simulink model "HANcoder_E407_TTA_Controller_v3_2"  (R2018b)
settings: Solver=FixedStepDiscrete  StartTime=0.0  StopTime=1  FixedStep=0.01  RelTol=1e-3
PreLoadFcn:
  | librarySetup
  | eval([bdroot,'_startup']) %Calling [modelName]_startup.m
undefined symbols (not defined in the file): A0, A1, A2, A3, A4, Backup_Board, basic_cycle_duration_bc0, basic_cycle_duration_bc1, comm_delay_estimation1, comm_delay_estimation2, COMM_Period, COMM_Phase1, COMM_Phase2, COMM_Phase_init1, COMM_Phase_init2, COMP_duration, CON2, CON4, Controller1_Board, Controller2_Board, Controller3_Board, D10, D12, D13, D8, D9, delta_a_set, delta_f_set, delta_max, delta_min, delta_precision, e_width, frequency_IRQ, HANtuneOverride, hardware_granularity, I_a, I_f, idle_time_init, Input_Gen_Board, LA_Clock_Gr, LA_COMM_dly, LA_COMM_Err, LA_E_Desync, LA_MEX_Flag, LA_Task_Act, m_v, Master_Role, matrix_cycle_duration, matrix_rows, max_desync, max_num_msgs_CAN1, max_num_msgs_CAN2, min_desync, OutControl1_ID, OutControl2_ID, OutEmulator_ID, R_al, R_ar, R_fl, R_fr ... (+80)
libraries: hdlsllib x434, HANcoder_STM32_Target x28, simulink x3, simulink_extras x1
(part 14 of 31)

== system HANcoder_E407_TTA_Controller_v3_2/HANcoder STM32 Target - E407-STM32 algorithm/TTA CAN System/TTA System/Matrix Cycle Manager/Controller Matrix Cycle/controller basic cycle 1/COMP Task - TMR/TMR_load_msgs_1 ==
  note: STEP 1 - Gather Output1 and Output2 messages
  note: Logic Analyzer - DEBUG
      | LT Update COMP task
      | activation
  note: Logic Analyzer - DEBUG
  Enable : EnablePort
  Bus Selector : BusSelector  OutputSignals=Buffer_2,Buffer_3,Buffer_4,Buffer_5,Buffer_6,Buffer_7
  Constant{9..12} (4 alike) : Constant  Value=torque_precision
  Constant8 : Constant  Priority=28  OutDataTypeStr=boolean
  Data Store Read : DataStoreRead  DataStoreName=output_control1_msg
  Data Store Write : DataStoreWrite  Priority=1  DataStoreName=tau_fr_out1
  Data Store Write1 : DataStoreWrite  Priority=2  DataStoreName=tau_fl_out1
  Data Store Write19 : DataStoreWrite  Priority=29  DataStoreName=Toggle_Pin_A0
  Data Store Write2 : DataStoreWrite  Priority=3  DataStoreName=tau_ar_out1
  Data Store Write3 : DataStoreWrite  Priority=4  DataStoreName=tau_al_out1
  Data Store Write4 : DataStoreWrite  Priority=5  DataStoreName=set_miss_out1
  Data Store Write5 : DataStoreWrite  Priority=6  DataStoreName=sensor_miss_out1
  uint8_2float : Subsystem
  uint8_2float1 : Subsystem
  uint8_2float2 : Subsystem
  uint8_2float3 : Subsystem
  wires:
  Data Store Read/1 -> Bus Selector/1
  Bus Selector/1 -> uint8_2float/2(value)  "<Buffer_2>"
  Bus Selector/2 -> uint8_2float1/2(value)  "<Buffer_3>"
  Bus Selector/3 -> uint8_2float2/2(value)  "<Buffer_4>"
  Bus Selector/4 -> uint8_2float3/2(value)  "<Buffer_5>"
  Bus Selector/5 -> Data Store Write4/1  "<Buffer_6>"
  Bus Selector/6 -> Data Store Write5/1  "<Buffer_7>"
  Constant8/1 -> Data Store Write19/1
  Constant9/1 -> uint8_2float/1(precision)
  uint8_2float/1(decoded) -> Data Store Write/1  "torque_fr_out1_s"
  Constant10/1 -> uint8_2float1/1(precision)
  Constant11/1 -> uint8_2float2/1(precision)
  Constant12/1 -> uint8_2float3/1(precision)
  uint8_2float1/1(decoded) -> Data Store Write1/1  "torque_fl_out1_s"
  uint8_2float2/1(decoded) -> Data Store Write2/1  "torque_ar_out1_s"
  uint8_2float3/1(decoded) -> Data Store Write3/1  "torque_al_out1_s"

== system HANcoder_E407_TTA_Controller_v3_2/HANcoder STM32 Target - E407-STM32 algorithm/TTA CAN System/TTA System/Matrix Cycle Manager/Controller Matrix Cycle/controller basic cycle 1/COMP Task - TMR/TMR_load_msgs_2 ==
  note: Logic Analyzer - DEBUG
  note: Logic Analyzer - DEBUG
      | LT Update COMP task
      | activation
  note: STEP 1 - Gather Output1 and Output2 messages
  Enable : EnablePort
  Bus Selector1 : BusSelector  OutputSignals=Buffer_2,Buffer_3,Buffer_4,Buffer_5,Buffer_6,Buffer_7
  Constant{13..16} (4 alike) : Constant  Value=torque_precision
  Constant8 : Constant  Priority=28  OutDataTypeStr=boolean
  Data Store Read1 : DataStoreRead  DataStoreName=output_control2_msg
  Data Store Write10 : DataStoreWrite  Priority=11  DataStoreName=set_miss_out2
  Data Store Write11 : DataStoreWrite  Priority=12  DataStoreName=sensor_miss_out2
  Data Store Write19 : DataStoreWrite  Priority=29  DataStoreName=Toggle_Pin_A0
  Data Store Write6 : DataStoreWrite  Priority=7  DataStoreName=tau_fr_out2
  Data Store Write7 : DataStoreWrite  Priority=8  DataStoreName=tau_fl_out2
  Data Store Write8 : DataStoreWrite  Priority=9  DataStoreName=tau_ar_out2
  Data Store Write9 : DataStoreWrite  Priority=10  DataStoreName=tau_al_out2
  uint8_2float4 : Subsystem
  uint8_2float5 : Subsystem
  uint8_2float6 : Subsystem
  uint8_2float7 : Subsystem
  wires:
  uint8_2float4/1(decoded) -> Data Store Write6/1  "torque_fr_out2_s"
  uint8_2float5/1(decoded) -> Data Store Write7/1  "torque_fl_out2_s"
  uint8_2float6/1(decoded) -> Data Store Write8/1  "torque_ar_out2_s"
  uint8_2float7/1(decoded) -> Data Store Write9/1  "torque_al_out2_s"
  Constant16/1 -> uint8_2float7/1(precision)
  Constant15/1 -> uint8_2float6/1(precision)
  Constant14/1 -> uint8_2float5/1(precision)
  Bus Selector1/1 -> uint8_2float4/2(value)  "<Buffer_2>"
  Constant13/1 -> uint8_2float4/1(precision)
  Constant8/1 -> Data Store Write19/1
  Data Store Read1/1 -> Bus Selector1/1
  Bus Selector1/2 -> uint8_2float5/2(value)  "<Buffer_3>"
  Bus Selector1/3 -> uint8_2float6/2(value)  "<Buffer_4>"
  Bus Selector1/4 -> uint8_2float7/2(value)  "<Buffer_5>"
  Bus Selector1/5 -> Data Store Write10/1  "<Buffer_6>"
  Bus Selector1/6 -> Data Store Write11/1  "<Buffer_7>"

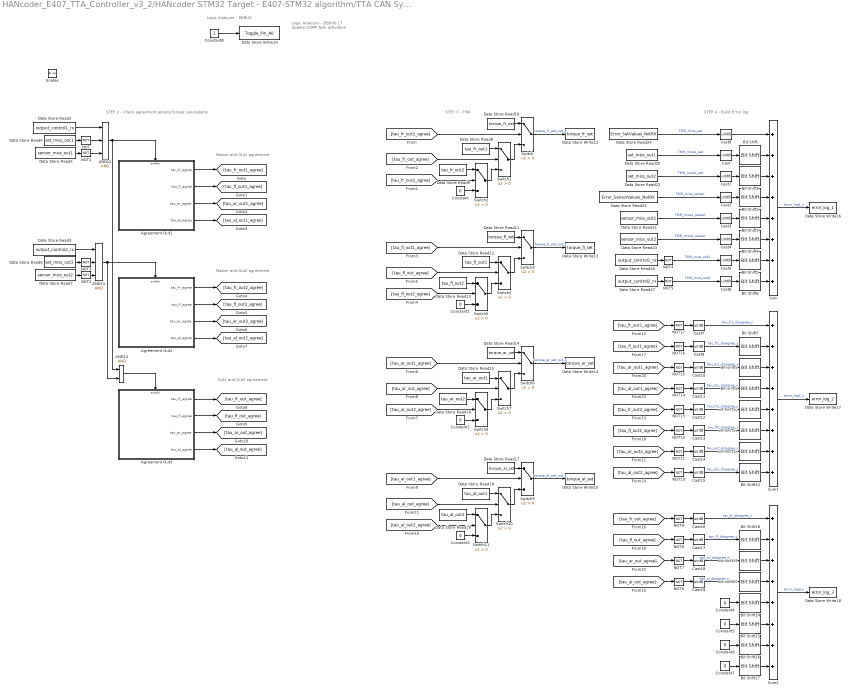
== system HANcoder_E407_TTA_Controller_v3_2/HANcoder STM32 Target - E407-STM32 algorithm/TTA CAN System/TTA System/Matrix Cycle Manager/Controller Matrix Cycle/controller basic cycle 1/COMP Task - TMR/TMR_main ==
  note: Master and Out1 agreement
  note: Logic Analyzer - DEBUG
  note: Logic Analyzer - DEBUG
      | LT Update COMP task
      | activation
  note: STEP 2 - Check agreement among torque calculations
  note: STEP 3 - TMR
  note: STEP 4 - Build Error log
  note: Master and Out2 agreement
  note: Out1 and Out2 agreement
  Enable : EnablePort
  AND12 : Logic  Inputs=3  IconShape=distinctive  AllPortsSameDT=off  OutDataTypeStr=boolean
  AND13 : Logic  Inputs=3  IconShape=distinctive  AllPortsSameDT=off  OutDataTypeStr=boolean
  AND14 : Logic  IconShape=distinctive  AllPortsSameDT=off  OutDataTypeStr=boolean
  Agreement Out1 : Subsystem  Priority=20  TreatAsAtomicUnit=on
  Agreement Out2 : Subsystem  Priority=21  TreatAsAtomicUnit=on
  Agreement Out3 : Subsystem  Priority=22  TreatAsAtomicUnit=on
  Bit Shift : hdlsllib/Logic and Bit Operations/Bit Shift  mode=Shift Left Logical  N=1
      settings: SourceProductName=HDL Coder  SourceProductBaseCode=HD
  Bit Shift1 : hdlsllib/Logic and Bit Operations/Bit Shift  mode=Shift Left Logical  N=2
      settings: SourceProductName=HDL Coder  SourceProductBaseCode=HD
  Bit Shift10 : hdlsllib/Logic and Bit Operations/Bit Shift  mode=Shift Left Logical  N=4
      settings: SourceProductName=HDL Coder  SourceProductBaseCode=HD
  Bit Shift11 : hdlsllib/Logic and Bit Operations/Bit Shift  mode=Shift Left Logical  N=5
      settings: SourceProductName=HDL Coder  SourceProductBaseCode=HD
  Bit Shift12 : hdlsllib/Logic and Bit Operations/Bit Shift  mode=Shift Left Logical  N=6
      settings: SourceProductName=HDL Coder  SourceProductBaseCode=HD
  Bit Shift13 : hdlsllib/Logic and Bit Operations/Bit Shift  mode=Shift Left Logical  N=7
      settings: SourceProductName=HDL Coder  SourceProductBaseCode=HD
  Bit Shift14 : hdlsllib/Logic and Bit Operations/Bit Shift  mode=Shift Left Logical  N=4
      settings: SourceProductName=HDL Coder  SourceProductBaseCode=HD
  Bit Shift15 : hdlsllib/Logic and Bit Operations/Bit Shift  mode=Shift Left Logical  N=5
      settings: SourceProductName=HDL Coder  SourceProductBaseCode=HD
  Bit Shift16 : hdlsllib/Logic and Bit Operations/Bit Shift  mode=Shift Left Logical  N=6
      settings: SourceProductName=HDL Coder  SourceProductBaseCode=HD
  Bit Shift17 : hdlsllib/Logic and Bit Operations/Bit Shift  mode=Shift Left Logical  N=7
      settings: SourceProductName=HDL Coder  SourceProductBaseCode=HD
  Bit Shift18 : hdlsllib/Logic and Bit Operations/Bit Shift  mode=Shift Left Logical  N=1
      settings: SourceProductName=HDL Coder  SourceProductBaseCode=HD
  Bit Shift19 : hdlsllib/Logic and Bit Operations/Bit Shift  mode=Shift Left Logical  N=2
      settings: SourceProductName=HDL Coder  SourceProductBaseCode=HD
  Bit Shift2 : hdlsllib/Logic and Bit Operations/Bit Shift  mode=Shift Left Logical  N=3
      settings: SourceProductName=HDL Coder  SourceProductBaseCode=HD
  Bit Shift20 : hdlsllib/Logic and Bit Operations/Bit Shift  mode=Shift Left Logical  N=3
      settings: SourceProductName=HDL Coder  SourceProductBaseCode=HD
  Bit Shift3 : hdlsllib/Logic and Bit Operations/Bit Shift  mode=Shift Left Logical  N=4
      settings: SourceProductName=HDL Coder  SourceProductBaseCode=HD
  Bit Shift4 : hdlsllib/Logic and Bit Operations/Bit Shift  mode=Shift Left Logical  N=5
      settings: SourceProductName=HDL Coder  SourceProductBaseCode=HD
  Bit Shift5 : hdlsllib/Logic and Bit Operations/Bit Shift  mode=Shift Left Logical  N=6
      settings: SourceProductName=HDL Coder  SourceProductBaseCode=HD
  Bit Shift6 : hdlsllib/Logic and Bit Operations/Bit Shift  mode=Shift Left Logical  N=7
      settings: SourceProductName=HDL Coder  SourceProductBaseCode=HD
  Bit Shift7 : hdlsllib/Logic and Bit Operations/Bit Shift  mode=Shift Left Logical  N=1
      settings: SourceProductName=HDL Coder  SourceProductBaseCode=HD
  Bit Shift8 : hdlsllib/Logic and Bit Operations/Bit Shift  mode=Shift Left Logical  N=2
      settings: SourceProductName=HDL Coder  SourceProductBaseCode=HD
  Bit Shift9 : hdlsllib/Logic and Bit Operations/Bit Shift  mode=Shift Left Logical  N=3
      settings: SourceProductName=HDL Coder  SourceProductBaseCode=HD
  Cast{,1..19} (20 alike) : DataTypeConversion  OutDataTypeStr=uint8
  Constant{,1..7} (8 alike) : Constant  Value=0  OutDataTypeStr=uint8
  Constant8 : Constant  Priority=28  OutDataTypeStr=boolean
  Data Store Read10 : DataStoreRead  DataStoreName=torque_fr_set
  Data Store Read11 : DataStoreRead  DataStoreName=torque_fl_set
  Data Store Read12 : DataStoreRead  DataStoreName=tau_fl_out1
  Data Store Read13 : DataStoreRead  DataStoreName=tau_fl_out2
  Data Store Read14 : DataStoreRead  DataStoreName=torque_ar_set
  Data Store Read15 : DataStoreRead  DataStoreName=tau_ar_out1
  Data Store Read16 : DataStoreRead  DataStoreName=tau_ar_out2
  Data Store Read17 : DataStoreRead  DataStoreName=torque_al_set
  Data Store Read18 : DataStoreRead  DataStoreName=tau_al_out1
  Data Store Read19 : DataStoreRead  DataStoreName=tau_al_out2
  Data Store Read2 : DataStoreRead  DataStoreName=output_control1_rx
  Data Store Read20 : DataStoreRead  DataStoreName=set_miss_out1
  Data Store Read21 : DataStoreRead  DataStoreName=sensor_miss_out1
  Data Store Read22 : DataStoreRead  DataStoreName=set_miss_out2
  Data Store Read23 : DataStoreRead  DataStoreName=sensor_miss_out2
  Data Store Read24 : DataStoreRead  DataStoreName=Error_SetValues_NotRX
  Data Store Read25 : DataStoreRead  DataStoreName=Error_SensorValues_NotRX
  Data Store Read26 : DataStoreRead  DataStoreName=output_control1_rx
  Data Store Read27 : DataStoreRead  DataStoreName=output_control2_rx
  Data Store Read3 : DataStoreRead  DataStoreName=output_control2_rx
  Data Store Read4 : DataStoreRead  DataStoreName=set_miss_out1
  Data Store Read5 : DataStoreRead  DataStoreName=sensor_miss_out1
  Data Store Read6 : DataStoreRead  DataStoreName=set_miss_out2
  Data Store Read7 : DataStoreRead  DataStoreName=sensor_miss_out2
  Data Store Read8 : DataStoreRead  DataStoreName=tau_fr_out1
  Data Store Read9 : DataStoreRead  DataStoreName=tau_fr_out2
  Data Store Write12 : DataStoreWrite  Priority=30  DataStoreName=torque_fr_set
  Data Store Write13 : DataStoreWrite  Priority=31  DataStoreName=torque_fl_set
  Data Store Write14 : DataStoreWrite  Priority=32  DataStoreName=torque_ar_set
  Data Store Write15 : DataStoreWrite  Priority=33  DataStoreName=torque_al_set
  Data Store Write16 : DataStoreWrite  Priority=50  DataStoreName=error_log_1
  Data Store Write17 : DataStoreWrite  Priority=51  DataStoreName=error_log_2
  Data Store Write18 : DataStoreWrite  Priority=52  DataStoreName=error_log_3
  Data Store Write19 : DataStoreWrite  Priority=29  DataStoreName=Toggle_Pin_A0
  NOT{,1..17} (18 alike) : Logic  Operator=NOT  IconShape=distinctive  AllPortsSameDT=off  OutDataTypeStr=boolean
  Sum : Sum  Priority=40  Inputs=++++++++
  Sum1 : Sum  Priority=41  Inputs=++++++++
  Sum2 : Sum  Priority=42  Inputs=++++++++
  Switch{,1..11} (12 alike) : Switch  Criteria=u2 > Threshold
  wires:
  Cast19/1 -> Bit Shift20/1  "tau_al_disagree_s"
  Cast18/1 -> Bit Shift19/1  "tau_ar_disagree_s"
  Cast17/1 -> Bit Shift18/1  "tau_fl_disagree_s"
  Cast16/1 -> Sum2/1  "tau_fr_disagree_s"
  Cast15/1 -> Bit Shift13/1  "tau_al2_disagree_s"
  Cast14/1 -> Bit Shift12/1  "tau_ar2_disagree_s"
  Cast13/1 -> Bit Shift11/1  "tau_fl2_disagree_s"
  Cast12/1 -> Bit Shift10/1  "tau_fr2_disagree_s"
  Cast11/1 -> Bit Shift9/1  "tau_al1_disagree_s"
  Cast10/1 -> Bit Shift8/1  "tau_ar1_disagree_s"
  Cast9/1 -> Bit Shift7/1  "tau_fl1_disagree_s"
  Cast8/1 -> Sum/1
  Cast7/1 -> Sum1/1  "tau_fr1_disagree_s"
  Cast6/1 -> Bit Shift6/1
  Cast5/1 -> Bit Shift5/1
  Cast4/1 -> Bit Shift4/1
  Cast3/1 -> Bit Shift3/1
  Cast2/1 -> Bit Shift2/1
  Cast1/1 -> Bit Shift1/1
  Cast/1 -> Bit Shift/1
  Constant8/1 -> Data Store Write19/1
  Constant5/1 -> Bit Shift15/1
  Constant6/1 -> Bit Shift16/1
  Constant7/1 -> Bit Shift17/1
  Constant4/1 -> Bit Shift14/1
  [tau_al_out_agree] -> NOT6/1
  [tau_ar_out_agree] -> NOT7/1
  [tau_fl_out_agree] -> NOT8/1
  [tau_fr_out_agree] -> NOT9/1
  [tau_al_out2_agree] -> NOT10/1
  [tau_ar_out2_agree] -> NOT11/1
  [tau_fl_out2_agree] -> NOT12/1
  [tau_fr_out1_agree] -> NOT17/1
  [tau_fr_out2_agree] -> NOT13/1
  [tau_al_out1_agree] -> NOT14/1
  [tau_ar_out1_agree] -> NOT15/1
  [tau_fl_out1_agree] -> NOT16/1
  Bit Shift17/1 -> Sum2/8
  Bit Shift16/1 -> Sum2/7
  Bit Shift15/1 -> Sum2/6
  Bit Shift14/1 -> Sum2/5
  Bit Shift20/1 -> Sum2/4
  Bit Shift19/1 -> Sum2/3
  Bit Shift13/1 -> Sum1/8
  Bit Shift12/1 -> Sum1/7
  Bit Shift11/1 -> Sum1/6
  Bit Shift10/1 -> Sum1/5
  Bit Shift9/1 -> Sum1/4
  Bit Shift8/1 -> Sum1/3
  Bit Shift18/1 -> Sum2/2
  Sum2/1 -> Data Store Write18/1  "error_log3_s"
  Bit Shift7/1 -> Sum1/2
  Sum1/1 -> Data Store Write17/1  "error_log2_s"
  NOT5/1 -> Cast6/1  "TMR_miss_out2"
  NOT4/1 -> Cast5/1  "TMR_miss_out1"
  Data Store Read27/1 -> NOT5/1
  Data Store Read26/1 -> NOT4/1
  Data Store Read21/1 -> Cast3/1  "TMR_miss1_sensor"
  Data Store Read23/1 -> Cast4/1  "TMR_miss2_sensor"
  Data Store Read25/1 -> Cast2/1  "TMR_miss_sensor"
  Bit Shift6/1 -> Sum/8
  Bit Shift5/1 -> Sum/7
  Bit Shift4/1 -> Sum/6
  Bit Shift3/1 -> Sum/5
  Bit Shift2/1 -> Sum/4
  Sum/1 -> Data Store Write16/1  "error_log1_s"
  Data Store Read22/1 -> Cast1/1  "TMR_miss2_set"
  Data Store Read20/1 -> Cast/1  "TMR_miss1_set"
  Data Store Read24/1 -> Cast8/1  "TMR_miss_set"
  Bit Shift1/1 -> Sum/3
  Bit Shift/1 -> Sum/2
  AND14/1 -> Agreement Out3/Enable
  NOT2/1 -> AND13/3
  NOT3/1 -> AND13/2
  AND13/1 -> Agreement Out2/Enable, AND14/2
  Data Store Read7/1 -> NOT2/1
  Data Store Read6/1 -> NOT3/1
  Data Store Read3/1 -> AND13/1
  Data Store Read2/1 -> AND12/1
  NOT/1 -> AND12/2
  NOT1/1 -> AND12/3
  AND12/1 -> Agreement Out1/Enable, AND14/1
  Data Store Read5/1 -> NOT1/1
  Data Store Read4/1 -> NOT/1
  Switch10/1 -> Switch9/3
  Switch11/1 -> Switch10/3
  Data Store Read19/1 -> Switch11/1
  [tau_al_out_agree] -> Switch10/2
  [tau_al_out2_agree] -> Switch11/2
  [tau_al_out1_agree] -> Switch9/2
  Constant3/1 -> Switch11/3
  Data Store Read17/1 -> Switch9/1
  Data Store Read18/1 -> Switch10/1
  Switch9/1 -> Data Store Write15/1  "torque_al_set_out_s"
  Switch6/1 -> Data Store Write14/1  "torque_ar_set_out_s"
  Data Store Read15/1 -> Switch7/1
  Data Store Read14/1 -> Switch6/1
  Constant2/1 -> Switch8/3
  [tau_ar_out1_agree] -> Switch6/2
  [tau_ar_out2_agree] -> Switch8/2
  [tau_ar_out_agree] -> Switch7/2
  Data Store Read16/1 -> Switch8/1
  Switch8/1 -> Switch7/3
  Switch7/1 -> Switch6/3
  Switch4/1 -> Switch3/3
  Switch5/1 -> Switch4/3
  Data Store Read13/1 -> Switch5/1
  [tau_fl_out_agree] -> Switch4/2
  [tau_fl_out2_agree] -> Switch5/2
  [tau_fl_out1_agree] -> Switch3/2
  Constant1/1 -> Switch5/3
  Data Store Read11/1 -> Switch3/1
  Data Store Read12/1 -> Switch4/1
  Switch3/1 -> Data Store Write13/1  "torque_fl_set_out_s"
  Switch/1 -> Data Store Write12/1  "torque_fr_set_out_s"
  Data Store Read8/1 -> Switch1/1
  Data Store Read10/1 -> Switch/1
  Constant/1 -> Switch2/3
  [tau_fr_out1_agree] -> Switch/2
  [tau_fr_out2_agree] -> Switch2/2
  [tau_fr_out_agree] -> Switch1/2
  Data Store Read9/1 -> Switch2/1
  Switch2/1 -> Switch1/3
  Switch1/1 -> Switch/3
  Agreement Out3/4(tau_al_agree) -> [tau_al_out_agree]
  Agreement Out3/3(tau_ar_agree) -> [tau_ar_out_agree]
  Agreement Out3/2("tau_fl_agree ") -> [tau_fl_out_agree]
  Agreement Out3/1(tau_fr_agree) -> [tau_fr_out_agree]
  Agreement Out2/4(tau_al_agree) -> [tau_al_out2_agree]
  Agreement Out2/3(tau_ar_agree) -> [tau_ar_out2_agree]
  Agreement Out2/2("tau_fl_agree ") -> [tau_fl_out2_agree]
  Agreement Out2/1(tau_fr_agree) -> [tau_fr_out2_agree]
  Agreement Out1/4(tau_al_agree) -> [tau_al_out1_agree]
  Agreement Out1/3(tau_ar_agree) -> [tau_ar_out1_agree]
  Agreement Out1/2("tau_fl_agree ") -> [tau_fl_out1_agree]
  Agreement Out1/1(tau_fr_agree) -> [tau_fr_out1_agree]
  NOT6/1 -> Cast19/1
  NOT7/1 -> Cast18/1
  NOT8/1 -> Cast17/1
  NOT9/1 -> Cast16/1
  NOT10/1 -> Cast15/1
  NOT11/1 -> Cast14/1
  NOT12/1 -> Cast13/1
  NOT13/1 -> Cast12/1
  NOT14/1 -> Cast11/1
  NOT15/1 -> Cast10/1
  NOT16/1 -> Cast9/1
  NOT17/1 -> Cast7/1

== system HANcoder_E407_TTA_Controller_v3_2/HANcoder STM32 Target - E407-STM32 algorithm/TTA CAN System/TTA System/Matrix Cycle Manager/Controller Matrix Cycle/controller basic cycle 1/COMP Task - Update LT1/LA - Ensemble precision ==
  note: Logic Analyzer - DEBUG
      | Ensemble precision
      | measurement (Desync)
  Enable : EnablePort
  Constant2 : Constant  Priority=28  OutDataTypeStr=boolean
  Data Store Write1 : DataStoreWrite  Priority=29  DataStoreName=Toggle_Pin_D10
  wires:
  Constant2/1 -> Data Store Write1/1

== system HANcoder_E407_TTA_Controller_v3_2/HANcoder STM32 Target - E407-STM32 algorithm/TTA CAN System/TTA System/Matrix Cycle Manager/Controller Matrix Cycle/controller basic cycle 1/COMP Task - Update LT1/Local Time Update ==
  note: If the desync is negative, the Local Time
      | gets updated straight away. Otherwise,
      | the Local Time must be updated in small
      | steps.
  note: Desync Check
  note: Local Time Update Acknowledge
  note: Global - Local time update acknowledge
  note: Logic Analyzer - DEBUG
      | LT Update COMP task
      | activation
  note: Logic Analyzer - DEBUG
  note: Logic Analyzer - DEBUG
      | Ensemble precision
      | measurement (Desync)
  Time_Mark : Inport
  Enable : EnablePort
  Constant1 : Constant  Priority=28  OutDataTypeStr=boolean
  Constant2 : Constant  Priority=28  OutDataTypeStr=boolean
  Constant3 : Constant  Priority=24  OutDataTypeStr=boolean
  Constant4 : Constant  Value=0
  Data Store Read1 : DataStoreRead  Priority=11  DataStoreName=Desync_Ticks
  Data Store Write : DataStoreWrite  DataStoreName=Desync_Positive
  Data Store Write1 : DataStoreWrite  Priority=29  DataStoreName=Toggle_Pin_D10
  Data Store Write13 : DataStoreWrite  Priority=25  DataStoreName=BC1_Sync_processed
  Data Store Write3 : DataStoreWrite  Priority=29  DataStoreName=Toggle_Pin_A0
  Desync_Negative : Subsystem  TreatAsAtomicUnit=on
  GreaterThan : RelationalOperator  Operator=>  OutDataTypeStr=boolean  RndMeth=Simplest
  NOT : Logic  Operator=NOT  IconShape=distinctive  AllPortsSameDT=off  OutDataTypeStr=boolean
  wires:
  Constant1/1 -> Data Store Write3/1
  Constant3/1 -> Data Store Write13/1
  Data Store Read1/1 -> GreaterThan/1
  Constant4/1 -> GreaterThan/2
  NOT/1 -> Desync_Negative/Enable
  GreaterThan/1 -> NOT/1, Data Store Write/1
  Time_Mark/1 -> Desync_Negative/1(Current_Local_Time)
  Constant2/1 -> Data Store Write1/1

== system HANcoder_E407_TTA_Controller_v3_2/HANcoder STM32 Target - E407-STM32 algorithm/TTA CAN System/TTA System/Matrix Cycle Manager/Input Generator Matrix Cycle/input generator basic cycle 0/COMM Task - Sync bc 0/Reception substasks ==
  note: After the beginning of the task
  note: LT > TM_COMM
  note: LT == TM_COMM
  note: Beginning of the task
  note: Still no msg received
  Time_Mark : Inport
  RX_ID : Inport  Port=2
  Enable : EnablePort
  AND : Logic  IconShape=distinctive  AllPortsSameDT=off  OutDataTypeStr=boolean
  AND1 : Logic  IconShape=distinctive  AllPortsSameDT=off  OutDataTypeStr=boolean
  Data Store Read : DataStoreRead  DataStoreName=Local_Ticks
  Data Store Read1 : DataStoreRead  DataStoreName=New_Msg_Ready_CAN1
  Data Store Read2 : DataStoreRead  DataStoreName=New_Msg_Ready_CAN2
  Equal16 : RelationalOperator  Operator===  OutDataTypeStr=boolean  RndMeth=Simplest
  Equal2 : RelationalOperator  Operator=>  OutDataTypeStr=boolean  RndMeth=Simplest
  NOT : Logic  Operator=NOT  IconShape=distinctive  AllPortsSameDT=off  OutDataTypeStr=boolean
  NOT1 : Logic  Operator=NOT  IconShape=distinctive  AllPortsSameDT=off  OutDataTypeStr=boolean
  RX buffers update : Subsystem  Priority=20
  Receive CAN1 : Outport  OutputWhenDisabled=reset  InitialOutput=0
  Receive CAN2 : Outport  Port=2  OutputWhenDisabled=reset  InitialOutput=0
  wires:
  AND1/1 -> Receive CAN2/1
  AND/1 -> Receive CAN1/1
  Equal2/1 -> AND/1, AND1/1
  NOT/1 -> AND/2
  NOT1/1 -> AND1/2
  Data Store Read2/1 -> NOT1/1
  Data Store Read1/1 -> NOT/1
  RX_ID/1 -> RX buffers update/1(Rx_ID)
  Equal16/1 -> RX buffers update/Enable
  Data Store Read/1 -> Equal16/1, Equal2/1
  Time_Mark/1 -> Equal16/2, Equal2/2

== system HANcoder_E407_TTA_Controller_v3_2/HANcoder STM32 Target - E407-STM32 algorithm/TTA CAN System/TTA System/Matrix Cycle Manager/Input Generator Matrix Cycle/input generator basic cycle 0/COMM Task - Sync bc 0/Transmission subtasks ==
  note: Encode value domain message at the start of the task
  note: Beginning of the task
  note: LT == TM_COMM
  note: LT > TM_COMM
  note: After the beginning of the task
  note: Check if we have not surpassed
      | maximum number of Tx messages
  note: Check if we have not surpassed
      | maximum number of Tx messages
  Time_Mark : Inport
  TX_ID : Inport  Port=2
  Enable : EnablePort
  AND : Logic  IconShape=distinctive  AllPortsSameDT=off  OutDataTypeStr=boolean
  AND1 : Logic  IconShape=distinctive  AllPortsSameDT=off  OutDataTypeStr=boolean
  Check msg transmission CAN1 : Subsystem
  Check msg transmission CAN2 : Subsystem
  Constant6 : Constant  Value=max_num_msgs_CAN1
  Constant7 : Constant  Value=max_num_msgs_CAN2
  Data Store Read : DataStoreRead  DataStoreName=Local_Ticks
  Data Store Read2 : DataStoreRead  DataStoreName=Tx_msg_count_CAN1
  Data Store Read3 : DataStoreRead  DataStoreName=Tx_msg_count_CAN2
  Equal16 : RelationalOperator  Operator===  OutDataTypeStr=boolean  RndMeth=Simplest
  Equal2 : RelationalOperator  Operator=>  OutDataTypeStr=boolean  RndMeth=Simplest
  GreaterThan2 : RelationalOperator  Operator=<=  OutDataTypeStr=boolean  RndMeth=Simplest
  GreaterThan3 : RelationalOperator  Operator=<=  OutDataTypeStr=boolean  RndMeth=Simplest
  Msg_Value_Data_Encoded : Subsystem
  Send CAN1 : Outport  OutputWhenDisabled=reset  InitialOutput=0
  Send CAN2 : Outport  Port=2  OutputWhenDisabled=reset  InitialOutput=0
  wires:
  Time_Mark/1 -> Check msg transmission CAN1/2(Time Mark), Check msg transmission CAN2/2(Time Mark), Equal2/2, Equal16/2
  Data Store Read/1 -> Check msg transmission CAN1/1(Local Time), Check msg transmission CAN2/1(Local Time), Equal2/1, Equal16/1
  Equal16/1 -> Msg_Value_Data_Encoded/Enable
  Check msg transmission CAN1/1(Send CAN1) -> Send CAN1/1
  Check msg transmission CAN2/1(Send CAN2) -> Send CAN2/1
  Data Store Read2/1 -> GreaterThan2/1
  Constant6/1 -> GreaterThan2/2
  Constant7/1 -> GreaterThan3/2
  Data Store Read3/1 -> GreaterThan3/1
  GreaterThan2/1 -> AND/2
  AND/1 -> Check msg transmission CAN1/Enable
  AND1/1 -> Check msg transmission CAN2/Enable
  GreaterThan3/1 -> AND1/2
  Msg_Value_Data_Encoded/1(Value_domain_msg) -> [Encoded_msg_TAG]
  [Encoded_msg_TAG] -> Check msg transmission CAN1/4(Value Domain Msg)
  [Encoded_msg_TAG] -> Check msg transmission CAN2/4(Value Domain Msg)
  TX_ID/1 -> [Tx_ID_TAG]
  [Tx_ID_TAG] -> Check msg transmission CAN1/3(Tx_ID)
  [Tx_ID_TAG] -> Check msg transmission CAN2/3(Tx_ID)
  Equal2/1 -> [Next_actions_TAG]
  [Next_actions_TAG] -> AND/1
  [Next_actions_TAG] -> AND1/1

== system HANcoder_E407_TTA_Controller_v3_2/HANcoder STM32 Target - E407-STM32 algorithm/TTA CAN System/TTA System/Matrix Cycle Manager/Input Generator Matrix Cycle/input generator basic cycle 0/COMP Task - Reset Board/Check Timeouts ==
  note: Timeout Master counter
  note: Logic Analyzer - DEBUG
  note: Logic Analyzer - DEBUG
      | Increase Error counter
  Enable : EnablePort
  Constant16 : Constant
  Data Store Read23 : DataStoreRead  DataStoreName=Sync_bc0_missed_counter
  Data Store Read24 : DataStoreRead  DataStoreName=Sync_bc0_missed_counter
  Data Store Read25 : DataStoreRead  DataStoreName=BC0_Sync_processed
  Data Store Write8 : DataStoreWrite  DataStoreName=Toggle_Pin_A1
  Data Store Write9 : DataStoreWrite  DataStoreName=Sync_bc0_missed_counter
  NOT4 : Logic  Operator=NOT  IconShape=distinctive  AllPortsSameDT=off  OutDataTypeStr=boolean
  Plus6 : Sum
  Switch7 : Switch  Criteria=u2 > Threshold
  wires:
  Constant16/1 -> Plus6/2
  Data Store Read23/1 -> Plus6/1
  Data Store Read24/1 -> Switch7/3
  Data Store Read25/1 -> NOT4/1
  Plus6/1 -> Switch7/1
  Switch7/1 -> Data Store Write9/1
  NOT4/1 -> Data Store Write8/1, Switch7/2

== system HANcoder_E407_TTA_Controller_v3_2/HANcoder STM32 Target - E407-STM32 algorithm/TTA CAN System/TTA System/Matrix Cycle Manager/Input Generator Matrix Cycle/input generator basic cycle 0/COMP Task - Reset Board/RESET Board - Return to initialization ==
  note: Logic Analyzer - DEBUG
  note: Logic Analyzer - DEBUG
      | Start of COMP task
  note: Reset board state
  note: CAN Rx preparation for sync
  note: Role reset
  Enable : EnablePort
  Cast : DataTypeConversion  OutDataTypeStr=boolean
  Cast6 : DataTypeConversion  OutDataTypeStr=uint8
  Constant : Constant  Value=0
  Constant1 : Constant  Value=Sync_ID  OutDataTypeStr=uint32
  Constant3 : Constant  OutDataTypeStr=boolean
  Data Store Write : DataStoreWrite  DataStoreName=Reset_Board
  Data Store Write1 : DataStoreWrite  DataStoreName=New_Msg_Ready_CAN1
  Data Store Write10 : DataStoreWrite  DataStoreName=New_Msg_Ready_CAN2
  Data Store Write11 : DataStoreWrite  DataStoreName=Desync_Positive
  Data Store Write2 : DataStoreWrite  DataStoreName=Initialization_flag
  Data Store Write3 : DataStoreWrite  DataStoreName=RxID_CAN1
  Data Store Write4 : DataStoreWrite  DataStoreName=Role_ID
  Data Store Write5 : DataStoreWrite  DataStoreName=Master_ID
  Data Store Write6 : DataStoreWrite  DataStoreName=Rx_State_CAN1
  Data Store Write7 : DataStoreWrite  DataStoreName=Toggle_Pin_A0
  Data Store Write8 : DataStoreWrite  DataStoreName=RxID_CAN2
  Data Store Write9 : DataStoreWrite  DataStoreName=Rx_State_CAN2
  NOT : Logic  Operator=NOT  IconShape=distinctive  AllPortsSameDT=off  OutDataTypeStr=boolean
  wires:
  Constant3/1 -> Data Store Write7/1
  Cast6/1 -> Data Store Write6/1, Data Store Write9/1
  Constant1/1 -> Data Store Write3/1, Data Store Write8/1
  NOT/1 -> Data Store Write2/1
  Cast/1 -> Data Store Write/1, NOT/1, Data Store Write11/1, Data Store Write1/1, Data Store Write10/1
  Constant/1 -> Cast/1, Cast6/1, Data Store Write4/1, Data Store Write5/1

== system HANcoder_E407_TTA_Controller_v3_2/HANcoder STM32 Target - E407-STM32 algorithm/TTA CAN System/TTA System/Matrix Cycle Manager/Input Generator Matrix Cycle/input generator basic cycle 0/COMP Task - Reset Variables BC0/Reset variables ==
  note: Logic Analyzer - DEBUG
  note: Logic Analyzer - DEBUG
      | Start of COMP task
  note: Reset variables
  Enable : EnablePort
  Constant : Constant  Value=0  OutDataTypeStr=boolean
  Constant3 : Constant  OutDataTypeStr=boolean
  Data Store Write : DataStoreWrite  DataStoreName=Desync_Positive
  Data Store Write1 : DataStoreWrite  DataStoreName=BC0_Sync_processed
  Data Store Write5 : DataStoreWrite  DataStoreName=Toggle_Pin_A0
  wires:
  Constant3/1 -> Data Store Write5/1
  Constant/1 -> Data Store Write/1, Data Store Write1/1

== system HANcoder_E407_TTA_Controller_v3_2/HANcoder STM32 Target - E407-STM32 algorithm/TTA CAN System/TTA System/Matrix Cycle Manager/Input Generator Matrix Cycle/input generator basic cycle 0/COMP Task - Sync bc0 check/Process_Messages ==
  note: Logic Analyzer - DEBUG
  note: Logic Analyzer - DEBUG
      | Sync_Check COMP task
      | activation
  new_CAN1_msg : Inport
  new_CAN2_msg : Inport  Port=2
  Rx_msg_CAN1 : Inport  Port=3  OutDataTypeStr=Bus: msg_buffer_type
  Rx_Msg_CAN2 : Inport  Port=4  OutDataTypeStr=Bus: msg_buffer_type
  expected_basic_cycle : Inport  Port=5
  TM_COMM : Inport  Port=6
  Enable : EnablePort
  Bus Selector : BusSelector  OutputSignals=signal1,Buffer_2,Buffer_3,Buffer_4,Buffer_5,Buffer_6,Buffer_7,Buffer_8
  Constant2 : Constant  Priority=28  OutDataTypeStr=boolean
  Data Store Write : DataStoreWrite  Priority=4  DataStoreName=Msg_Rx  DataStoreElements=Msg_Rx.Buffer_1#Msg_Rx.Buffer_2#Msg_Rx.Buffer_3#Msg_Rx.Buffer_4#Msg_Rx.Buffer_5#Msg_Rx.Buffer_6#Msg_Rx.Buffer_7#Msg_Rx.Buffer_8
  Data Store Write2 : DataStoreWrite  DataStoreName=new_msg_Rx
  Data Store Write3 : DataStoreWrite  Priority=29  DataStoreName=Toggle_Pin_A0
  Demux message CAN1 and check coherence : Subsystem  Priority=1
  Demux message CAN1 and check coherence1 : Subsystem  Priority=2
  Desync calculation : Subsystem  Priority=10
  OR : Logic  Operator=OR  IconShape=distinctive  AllPortsSameDT=off  OutDataTypeStr=boolean
  Switch : Switch  Priority=3  Criteria=u2 > Threshold
  wires:
  Bus Selector/8 -> Data Store Write/8  "<Buffer_8>"
  Bus Selector/7 -> Data Store Write/7  "<Buffer_7>"
  Bus Selector/6 -> Data Store Write/6  "<Buffer_6>"
  Bus Selector/5 -> Data Store Write/5  "<Buffer_5>"
  Bus Selector/4 -> Data Store Write/4  "<Buffer_4>"
  Bus Selector/3 -> Data Store Write/3  "<Buffer_3>"
  Bus Selector/2 -> Data Store Write/2  "<Buffer_2>"
  Bus Selector/1 -> Data Store Write/1  "<signal1>"
  Switch/1 -> Bus Selector/1
  Demux message CAN1 and check coherence1/2(Msg_Count_CAN2) -> [msg_count_CAN2]
  Demux message CAN1 and check coherence/2(Msg_Count_CAN1) -> [msg_count_CAN1]
  Constant2/1 -> Data Store Write3/1
  expected_basic_cycle/1 -> Demux message CAN1 and check coherence/2(expected_basic_cycle), Demux message CAN1 and check coherence1/2(expected_basic_cycle)
  Demux message CAN1 and check coherence1/3(CAN2_msg) -> Switch/3
  Demux message CAN1 and check coherence1/1(CAN2_msg_coherent) -> OR/2
  Demux message CAN1 and check coherence/1(CAN1_msg) -> Switch/1
  Rx_Msg_CAN2/1 -> Demux message CAN1 and check coherence1/1(CAN2_Rx_msg)
  Rx_msg_CAN1/1 -> Demux message CAN1 and check coherence/1(CAN1_Rx_msg)
  new_CAN2_msg/1 -> Demux message CAN1 and check coherence1/Enable
  new_CAN1_msg/1 -> Demux message CAN1 and check coherence/Enable
  [CAN1_msg_coherent_TAG] -> Desync calculation/2(New_msg_CAN1)
  Demux message CAN1 and check coherence/3(CAN1_msg_coherent) -> Switch/2, [CAN1_msg_coherent_TAG], OR/1
  [new_msg_Rx_TAG] -> Desync calculation/Enable
  OR/1 -> [new_msg_Rx_TAG], Data Store Write2/1
  TM_COMM/1 -> Desync calculation/1(TM_COMM)
  [msg_count_CAN2] -> Desync calculation/4(msg_count_CAN2)
  [msg_count_CAN1] -> Desync calculation/3(msg_count_CAN1)

== system HANcoder_E407_TTA_Controller_v3_2/HANcoder STM32 Target - E407-STM32 algorithm/TTA CAN System/TTA System/Matrix Cycle Manager/Input Generator Matrix Cycle/input generator basic cycle 0/COMP Task - Sync bc0 check/Reset Tx msg counter ==
  Enable : EnablePort
  Constant1 : Constant  Priority=2
  Constant6 : Constant  Priority=2
  Data Store Write1 : DataStoreWrite  Priority=4  DataStoreName=Tx_msg_count_CAN1
  Data Store Write2 : DataStoreWrite  Priority=4  DataStoreName=Tx_msg_count_CAN2
  wires:
  Constant1/1 -> Data Store Write2/1
  Constant6/1 -> Data Store Write1/1

== system HANcoder_E407_TTA_Controller_v3_2/HANcoder STM32 Target - E407-STM32 algorithm/TTA CAN System/TTA System/Matrix Cycle Manager/Input Generator Matrix Cycle/input generator basic cycle 0/COMP Task - Update LT/LA - Ensemble precision ==
  note: Logic Analyzer - DEBUG
      | Ensemble precision
      | measurement (Desync)
  Enable : EnablePort
  Constant2 : Constant  Priority=28  OutDataTypeStr=boolean
  Data Store Write1 : DataStoreWrite  Priority=29  DataStoreName=Toggle_Pin_D10
  wires:
  Constant2/1 -> Data Store Write1/1

== system HANcoder_E407_TTA_Controller_v3_2/HANcoder STM32 Target - E407-STM32 algorithm/TTA CAN System/TTA System/Matrix Cycle Manager/Input Generator Matrix Cycle/input generator basic cycle 0/COMP Task - Update LT/Local Time Update ==
  note: Logic Analyzer - DEBUG
  note: Logic Analyzer - DEBUG
      | LT Update COMP task
      | activation
  note: Global - Local time update acknowledge
  note: Local Time Update Acknowledge
  note: Desync Check
  note: If the desync is negative, the Local Time
      | gets updated straight away. Otherwise,
      | the Local Time must be updated in small
      | steps.
  note: Logic Analyzer - DEBUG
      | Ensemble precision
      | measurement (Desync)
  Time_Mark : Inport
  Enable : EnablePort
  Constant1 : Constant  Priority=28  OutDataTypeStr=boolean
  Constant2 : Constant  Priority=28  OutDataTypeStr=boolean
  Constant3 : Constant  Priority=24  OutDataTypeStr=boolean
  Constant4 : Constant  Value=0
  Data Store Read1 : DataStoreRead  Priority=11  DataStoreName=Desync_Ticks
  Data Store Write : DataStoreWrite  DataStoreName=Desync_Positive
  Data Store Write1 : DataStoreWrite  Priority=29  DataStoreName=Toggle_Pin_D10
  Data Store Write13 : DataStoreWrite  Priority=25  DataStoreName=BC0_Sync_processed
  Data Store Write3 : DataStoreWrite  Priority=29  DataStoreName=Toggle_Pin_A0
  Desync_Negative : Subsystem  TreatAsAtomicUnit=on
  GreaterThan : RelationalOperator  Operator=>  OutDataTypeStr=boolean  RndMeth=Simplest
  NOT : Logic  Operator=NOT  IconShape=distinctive  AllPortsSameDT=off  OutDataTypeStr=boolean
  wires:
  Time_Mark/1 -> Desync_Negative/1(Current_Local_Time)
  GreaterThan/1 -> Data Store Write/1, NOT/1
  NOT/1 -> Desync_Negative/Enable
  Constant4/1 -> GreaterThan/2
  Data Store Read1/1 -> GreaterThan/1
  Constant3/1 -> Data Store Write13/1
  Constant1/1 -> Data Store Write3/1
  Constant2/1 -> Data Store Write1/1

== system HANcoder_E407_TTA_Controller_v3_2/HANcoder STM32 Target - E407-STM32 algorithm/TTA CAN System/TTA System/Matrix Cycle Manager/Input Generator Matrix Cycle/input generator basic cycle 0/COMP Task - Update LT/Set Reset Board ==
  note: If no sync was received, reset the Input Generator
  Enable : EnablePort
  Constant : Constant  OutDataTypeStr=boolean
  Data Store Write : DataStoreWrite  DataStoreName=Reset_Board
  wires:
  Constant/1 -> Data Store Write/1

== system HANcoder_E407_TTA_Controller_v3_2/HANcoder STM32 Target - E407-STM32 algorithm/TTA CAN System/TTA System/Matrix Cycle Manager/Input Generator Matrix Cycle/input generator basic cycle 1/COMM Task - Set_Values/Reception substasks ==
  note: Still no msg received
  note: Beginning of the task
  note: LT == TM_COMM
  note: LT > TM_COMM
  note: After the beginning of the task
  Time_Mark : Inport
  RX_ID : Inport  Port=2
  Enable : EnablePort
  AND : Logic  IconShape=distinctive  AllPortsSameDT=off  OutDataTypeStr=boolean
  AND1 : Logic  IconShape=distinctive  AllPortsSameDT=off  OutDataTypeStr=boolean
  Data Store Read : DataStoreRead  DataStoreName=Local_Ticks
  Data Store Read1 : DataStoreRead  DataStoreName=New_Msg_Ready_CAN1
  Data Store Read2 : DataStoreRead  DataStoreName=New_Msg_Ready_CAN2
  Equal16 : RelationalOperator  Operator===  OutDataTypeStr=boolean  RndMeth=Simplest
  Equal2 : RelationalOperator  Operator=>  OutDataTypeStr=boolean  RndMeth=Simplest
  NOT : Logic  Operator=NOT  IconShape=distinctive  AllPortsSameDT=off  OutDataTypeStr=boolean
  NOT1 : Logic  Operator=NOT  IconShape=distinctive  AllPortsSameDT=off  OutDataTypeStr=boolean
  RX buffers update : Subsystem  Priority=20
  Receive CAN1 : Outport  OutputWhenDisabled=reset  InitialOutput=0
  Receive CAN2 : Outport  Port=2  OutputWhenDisabled=reset  InitialOutput=0
  wires:
  Time_Mark/1 -> Equal2/2, Equal16/2
  Data Store Read/1 -> Equal2/1, Equal16/1
  Equal16/1 -> RX buffers update/Enable
  RX_ID/1 -> RX buffers update/1(Rx_ID)
  Data Store Read1/1 -> NOT/1
  Data Store Read2/1 -> NOT1/1
  NOT1/1 -> AND1/2
  NOT/1 -> AND/2
  Equal2/1 -> AND1/1, AND/1
  AND/1 -> Receive CAN1/1
  AND1/1 -> Receive CAN2/1

== system HANcoder_E407_TTA_Controller_v3_2/HANcoder STM32 Target - E407-STM32 algorithm/TTA CAN System/TTA System/Matrix Cycle Manager/Input Generator Matrix Cycle/input generator basic cycle 1/COMM Task - Set_Values/Transmission subtasks ==
  note: Encode value domain message at the start of the task
  note: Beginning of the task
  note: LT == TM_COMM
  note: LT > TM_COMM
  note: After the beginning of the task
  note: Check if we have not surpassed
      | maximum number of Tx messages
  note: Check if we have not surpassed
      | maximum number of Tx messages
  Time_Mark : Inport
  TX_ID : Inport  Port=2
  Enable : EnablePort
  AND : Logic  IconShape=distinctive  AllPortsSameDT=off  OutDataTypeStr=boolean
  AND1 : Logic  IconShape=distinctive  AllPortsSameDT=off  OutDataTypeStr=boolean
  Check msg transmission CAN1 : Subsystem
  Check msg transmission CAN2 : Subsystem
  Constant6 : Constant  Value=max_num_msgs_CAN1
  Constant7 : Constant  Value=max_num_msgs_CAN2
  Data Store Read : DataStoreRead  DataStoreName=Local_Ticks
  Data Store Read2 : DataStoreRead  DataStoreName=Tx_msg_count_CAN1
  Data Store Read3 : DataStoreRead  DataStoreName=Tx_msg_count_CAN2
  Equal16 : RelationalOperator  Operator===  OutDataTypeStr=boolean  RndMeth=Simplest
  Equal2 : RelationalOperator  Operator=>  OutDataTypeStr=boolean  RndMeth=Simplest
  GreaterThan2 : RelationalOperator  Operator=<=  OutDataTypeStr=boolean  RndMeth=Simplest
  GreaterThan3 : RelationalOperator  Operator=<=  OutDataTypeStr=boolean  RndMeth=Simplest
  Msg_Value_Data_Encoded : Subsystem
  Send CAN1 : Outport  OutputWhenDisabled=reset  InitialOutput=0
  Send CAN2 : Outport  Port=2  OutputWhenDisabled=reset  InitialOutput=0
  wires:
  Time_Mark/1 -> Check msg transmission CAN1/2(Time Mark), Check msg transmission CAN2/2(Time Mark), Equal2/2, Equal16/2
  Data Store Read/1 -> Check msg transmission CAN1/1(Local Time), Check msg transmission CAN2/1(Local Time), Equal2/1, Equal16/1
  Equal16/1 -> Msg_Value_Data_Encoded/Enable
  Check msg transmission CAN1/1(Send CAN1) -> Send CAN1/1
  Check msg transmission CAN2/1(Send CAN2) -> Send CAN2/1
  Data Store Read2/1 -> GreaterThan2/1
  Constant6/1 -> GreaterThan2/2
  Constant7/1 -> GreaterThan3/2
  Data Store Read3/1 -> GreaterThan3/1
  GreaterThan2/1 -> AND/2
  AND/1 -> Check msg transmission CAN1/Enable
  AND1/1 -> Check msg transmission CAN2/Enable
  GreaterThan3/1 -> AND1/2
  Msg_Value_Data_Encoded/1(Value_domain_msg) -> [Encoded_msg_TAG]
  [Encoded_msg_TAG] -> Check msg transmission CAN1/4(Value Domain Msg)
  [Encoded_msg_TAG] -> Check msg transmission CAN2/4(Value Domain Msg)
  TX_ID/1 -> [Tx_ID_TAG]
  [Tx_ID_TAG] -> Check msg transmission CAN1/3(Tx_ID)
  [Tx_ID_TAG] -> Check msg transmission CAN2/3(Tx_ID)
  Equal2/1 -> [Next_actions_TAG]
  [Next_actions_TAG] -> AND/1
  [Next_actions_TAG] -> AND1/1

== system HANcoder_E407_TTA_Controller_v3_2/HANcoder STM32 Target - E407-STM32 algorithm/TTA CAN System/TTA System/Matrix Cycle Manager/Input Generator Matrix Cycle/input generator basic cycle 1/COMM Task - Sync bc 1/Reception substasks ==
  note: After the beginning of the task
  note: LT > TM_COMM
  note: LT == TM_COMM
  note: Beginning of the task
  note: Still no msg received
  Time_Mark : Inport
  RX_ID : Inport  Port=2
  Enable : EnablePort
  AND : Logic  IconShape=distinctive  AllPortsSameDT=off  OutDataTypeStr=boolean
  AND1 : Logic  IconShape=distinctive  AllPortsSameDT=off  OutDataTypeStr=boolean
  Data Store Read : DataStoreRead  DataStoreName=Local_Ticks
  Data Store Read1 : DataStoreRead  DataStoreName=New_Msg_Ready_CAN1
  Data Store Read2 : DataStoreRead  DataStoreName=New_Msg_Ready_CAN2
  Equal16 : RelationalOperator  Operator===  OutDataTypeStr=boolean  RndMeth=Simplest
  Equal2 : RelationalOperator  Operator=>  OutDataTypeStr=boolean  RndMeth=Simplest
  NOT : Logic  Operator=NOT  IconShape=distinctive  AllPortsSameDT=off  OutDataTypeStr=boolean
  NOT1 : Logic  Operator=NOT  IconShape=distinctive  AllPortsSameDT=off  OutDataTypeStr=boolean
  RX buffers update : Subsystem  Priority=20
  Receive CAN1 : Outport  OutputWhenDisabled=reset  InitialOutput=0
  Receive CAN2 : Outport  Port=2  OutputWhenDisabled=reset  InitialOutput=0
  wires:
  AND1/1 -> Receive CAN2/1
  AND/1 -> Receive CAN1/1
  Equal2/1 -> AND/1, AND1/1
  NOT/1 -> AND/2
  NOT1/1 -> AND1/2
  Data Store Read2/1 -> NOT1/1
  Data Store Read1/1 -> NOT/1
  RX_ID/1 -> RX buffers update/1(Rx_ID)
  Equal16/1 -> RX buffers update/Enable
  Data Store Read/1 -> Equal16/1, Equal2/1
  Time_Mark/1 -> Equal16/2, Equal2/2

== system HANcoder_E407_TTA_Controller_v3_2/HANcoder STM32 Target - E407-STM32 algorithm/TTA CAN System/TTA System/Matrix Cycle Manager/Input Generator Matrix Cycle/input generator basic cycle 1/COMM Task - Sync bc 1/Transmission subtasks ==
  note: Encode value domain message at the start of the task
  note: Beginning of the task
  note: LT == TM_COMM
  note: LT > TM_COMM
  note: After the beginning of the task
  note: Check if we have not surpassed
      | maximum number of Tx messages
  note: Check if we have not surpassed
      | maximum number of Tx messages
  Time_Mark : Inport
  TX_ID : Inport  Port=2
  Enable : EnablePort
  AND : Logic  IconShape=distinctive  AllPortsSameDT=off  OutDataTypeStr=boolean
  AND1 : Logic  IconShape=distinctive  AllPortsSameDT=off  OutDataTypeStr=boolean
  Check msg transmission CAN1 : Subsystem
  Check msg transmission CAN2 : Subsystem
  Constant6 : Constant  Value=max_num_msgs_CAN1
  Constant7 : Constant  Value=max_num_msgs_CAN2
  Data Store Read : DataStoreRead  DataStoreName=Local_Ticks
  Data Store Read2 : DataStoreRead  DataStoreName=Tx_msg_count_CAN1
  Data Store Read3 : DataStoreRead  DataStoreName=Tx_msg_count_CAN2
  Equal16 : RelationalOperator  Operator===  OutDataTypeStr=boolean  RndMeth=Simplest
  Equal2 : RelationalOperator  Operator=>  OutDataTypeStr=boolean  RndMeth=Simplest
  GreaterThan2 : RelationalOperator  Operator=<=  OutDataTypeStr=boolean  RndMeth=Simplest
  GreaterThan3 : RelationalOperator  Operator=<=  OutDataTypeStr=boolean  RndMeth=Simplest
  Msg_Value_Data_Encoded : Subsystem
  Send CAN1 : Outport  OutputWhenDisabled=reset  InitialOutput=0
  Send CAN2 : Outport  Port=2  OutputWhenDisabled=reset  InitialOutput=0
  wires:
  Time_Mark/1 -> Check msg transmission CAN1/2(Time Mark), Check msg transmission CAN2/2(Time Mark), Equal2/2, Equal16/2
  Data Store Read/1 -> Check msg transmission CAN1/1(Local Time), Check msg transmission CAN2/1(Local Time), Equal2/1, Equal16/1
  Equal16/1 -> Msg_Value_Data_Encoded/Enable
  Check msg transmission CAN1/1(Send CAN1) -> Send CAN1/1
  Check msg transmission CAN2/1(Send CAN2) -> Send CAN2/1
  Data Store Read2/1 -> GreaterThan2/1
  Constant6/1 -> GreaterThan2/2
  Constant7/1 -> GreaterThan3/2
  Data Store Read3/1 -> GreaterThan3/1
  GreaterThan2/1 -> AND/2
  AND/1 -> Check msg transmission CAN1/Enable
  AND1/1 -> Check msg transmission CAN2/Enable
  GreaterThan3/1 -> AND1/2
  Msg_Value_Data_Encoded/1(Value_domain_msg) -> [Encoded_msg_TAG]
  [Encoded_msg_TAG] -> Check msg transmission CAN1/4(Value Domain Msg)
  [Encoded_msg_TAG] -> Check msg transmission CAN2/4(Value Domain Msg)
  TX_ID/1 -> [Tx_ID_TAG]
  [Tx_ID_TAG] -> Check msg transmission CAN1/3(Tx_ID)
  [Tx_ID_TAG] -> Check msg transmission CAN2/3(Tx_ID)
  Equal2/1 -> [Next_actions_TAG]
  [Next_actions_TAG] -> AND/1
  [Next_actions_TAG] -> AND1/1

== system HANcoder_E407_TTA_Controller_v3_2/HANcoder STM32 Target - E407-STM32 algorithm/TTA CAN System/TTA System/Matrix Cycle Manager/Input Generator Matrix Cycle/input generator basic cycle 1/COMP Task - Reset Board/Check Timeouts ==
  note: Timeout Master counter
  note: Logic Analyzer - DEBUG
  note: Logic Analyzer - DEBUG
      | Increase Error counter
  Enable : EnablePort
  Constant16 : Constant
  Data Store Read23 : DataStoreRead  DataStoreName=Sync_bc1_missed_counter
  Data Store Read24 : DataStoreRead  DataStoreName=Sync_bc1_missed_counter
  Data Store Read25 : DataStoreRead  DataStoreName=BC1_Sync_processed
  Data Store Write8 : DataStoreWrite  DataStoreName=Toggle_Pin_A1
  Data Store Write9 : DataStoreWrite  DataStoreName=Sync_bc1_missed_counter
  NOT4 : Logic  Operator=NOT  IconShape=distinctive  AllPortsSameDT=off  OutDataTypeStr=boolean
  Plus6 : Sum
  Switch7 : Switch  Criteria=u2 > Threshold
  wires:
  Constant16/1 -> Plus6/2
  Data Store Read23/1 -> Plus6/1
  Data Store Read24/1 -> Switch7/3
  Data Store Read25/1 -> NOT4/1
  Plus6/1 -> Switch7/1
  Switch7/1 -> Data Store Write9/1
  NOT4/1 -> Data Store Write8/1, Switch7/2

== system HANcoder_E407_TTA_Controller_v3_2/HANcoder STM32 Target - E407-STM32 algorithm/TTA CAN System/TTA System/Matrix Cycle Manager/Input Generator Matrix Cycle/input generator basic cycle 1/COMP Task - Reset Board/RESET Board - Return to initialization ==
  note: Logic Analyzer - DEBUG
  note: Logic Analyzer - DEBUG
      | Start of COMP task
  note: Reset board state
  note: CAN Rx preparation for sync
  note: Role reset
  Enable : EnablePort
  Cast : DataTypeConversion  OutDataTypeStr=boolean
  Cast6 : DataTypeConversion  OutDataTypeStr=uint8
  Constant : Constant  Value=0
  Constant1 : Constant  Value=Sync_ID  OutDataTypeStr=uint32
  Constant3 : Constant  OutDataTypeStr=boolean
  Data Store Write : DataStoreWrite  DataStoreName=Reset_Board
  Data Store Write1 : DataStoreWrite  DataStoreName=New_Msg_Ready_CAN1
  Data Store Write10 : DataStoreWrite  DataStoreName=New_Msg_Ready_CAN2
  Data Store Write11 : DataStoreWrite  DataStoreName=Desync_Positive
  Data Store Write12 : DataStoreWrite  DataStoreName=BC1_Sync_processed
  Data Store Write2 : DataStoreWrite  DataStoreName=Initialization_flag
  Data Store Write3 : DataStoreWrite  DataStoreName=RxID_CAN1
  Data Store Write4 : DataStoreWrite  DataStoreName=Role_ID
  Data Store Write5 : DataStoreWrite  DataStoreName=Master_ID
  Data Store Write6 : DataStoreWrite  DataStoreName=Rx_State_CAN1
  Data Store Write7 : DataStoreWrite  DataStoreName=Toggle_Pin_A0
  Data Store Write8 : DataStoreWrite  DataStoreName=RxID_CAN2
  Data Store Write9 : DataStoreWrite  DataStoreName=Rx_State_CAN2
  NOT : Logic  Operator=NOT  IconShape=distinctive  AllPortsSameDT=off  OutDataTypeStr=boolean
  wires:
  Constant3/1 -> Data Store Write7/1
  Cast6/1 -> Data Store Write6/1, Data Store Write9/1
  Constant1/1 -> Data Store Write3/1, Data Store Write8/1
  NOT/1 -> Data Store Write2/1
  Constant/1 -> Cast/1, Cast6/1, Data Store Write4/1, Data Store Write5/1
  Cast/1 -> Data Store Write12/1, Data Store Write1/1, Data Store Write10/1, Data Store Write11/1, NOT/1, Data Store Write/1

== system HANcoder_E407_TTA_Controller_v3_2/HANcoder STM32 Target - E407-STM32 algorithm/TTA CAN System/TTA System/Matrix Cycle Manager/Input Generator Matrix Cycle/input generator basic cycle 1/COMP Task - Reset Variables BC1/Reset Variables ==
  note: Logic Analyzer - DEBUG
  note: Logic Analyzer - DEBUG
      | Start of COMP task
  note: Reset variables
  Enable : EnablePort
  Constant : Constant  Value=0  OutDataTypeStr=boolean
  Constant3 : Constant  OutDataTypeStr=boolean
  Data Store Write : DataStoreWrite  DataStoreName=Desync_Positive
  Data Store Write1 : DataStoreWrite  DataStoreName=BC1_Sync_processed
  Data Store Write3 : DataStoreWrite  DataStoreName=Toggle_Pin_A0
  wires:
  Constant3/1 -> Data Store Write3/1
  Constant/1 -> Data Store Write/1, Data Store Write1/1

== system HANcoder_E407_TTA_Controller_v3_2/HANcoder STM32 Target - E407-STM32 algorithm/TTA CAN System/TTA System/Matrix Cycle Manager/Input Generator Matrix Cycle/input generator basic cycle 1/COMP Task - Rx_Set_Values_Check/Reset Tx msg counter ==
  Enable : EnablePort
  Constant1 : Constant  Priority=2
  Constant6 : Constant  Priority=2
  Data Store Write1 : DataStoreWrite  Priority=4  DataStoreName=Tx_msg_count_CAN1
  Data Store Write2 : DataStoreWrite  Priority=4  DataStoreName=Tx_msg_count_CAN2
  wires:
  Constant1/1 -> Data Store Write2/1
  Constant6/1 -> Data Store Write1/1
